simulink model "pid_tv_test2"  (R2016a)
settings: Solver=ode23tb  StartTime=0.0  StopTime=ti(end)  MaxStep=1e-3
InitFcn:
  | fp_sp_k = 12e3;
  | fp_sp_d = 1;
  | weights = 70/6;
  | joint_k = 0*180/pi;
  | joint_d = 0*180/pi;
  | fp_uj_dp_k = 500*180/pi;
  | fp_uj_dp_d = 1*180/pi;
  | fp_uj_ie_k = 500*180/pi;
  | fp_uj_ie_d = 1*180/pi;
values from neighbouring files (symbols this model uses):
  N = length(shin_angles_in.signals.values)    [GaitEmu_code.m]    (also in dy1.m; dy2.m; est_joint.m = size( [body1.trans body2.trans], 1 ); impcont.m)
  s = [-atan((t2.*3.379e-4+t3+t4.*t5.*4.401e-2)./(t4.*cos(q2)));-asin(t2.*1.4870979e-5+t3.*4.401e-2-t4.*t5)]    [FK_af.m]    (also in FK_footimp.m = [atan((ree2_1.*t2.*4.401e-2+ree2_2.*t4+ree2_3.*t3+t5.*t7.*4.; FK_gaitEmul.m = [q1+t2.*t4.*4.234e-1+t3.*t5.*1.5e-3-t2.*t6.*t7.*1.5e-3-5.347; ik.m = [x; y; z]; ik_af.m = FK_af(q))
  sta = [-0.5345 0.03779 -0.0866]    [GaitEmu_code.m]    (also in dy1.m; dy2.m; grn_dyn.m; impcont.m)
  Y = -( reshape( body1.trans', [], 1 ) - reshape( body2.trans', [], 1 ) )    [creat_joint.m]    (also in est_joint.m = -( reshape( body1.trans', [3*N 1] ) - reshape( body2.trans',)
undefined symbols (not defined in the file or in its folder): X, Z
libraries: sm_lib x263, nesl_utility x76, simulink x4, dspstat3 x1
(part 6 of 6)

== system pid_tv_test2/Gait Emulator/prismatic frame1/y_bar_w_weightWalk_Sim1_1_RIGID/weight_4_RIGID ==
  ReferenceFrame : sm_lib/Frames and Transforms/Reference Frame
  Solid : sm_lib/Body Elements/Solid  InertiaType=Custom  Mass=weights  MassUnits=kg  CenterOfMass=[-0.093540130299891208 0.042272178743630776 0.014999999999999999]  CenterOfMassUnits=m  MomentsOfInertia=[0.0088271162208858108 0.0088271162208858108 0.017393538113134353]  MomentsOfInertiaUnits=kg*m^2  ProductsOfInertia=[0 0 0]  ProductsOfInertiaUnits=kg*m^2  DensityBased=on  Density=1000  DensityUnits=kg/(m^3)  DoExposeReferenceFrame=on  SerializedFrames=<Frames/>  GraphicType=FromGeometry  MarkerShape=Sphere  MarkerSize=10  MarkerSizeUnits=m  GraphicVisPropType=SimpleVisualProperties  GraphicDiffuseColor=[0.792156862745098 0.81960784313725488 0.93333333333333335]  GraphicSpecularColor=[0.5 0.5 0.5 1.0]  GraphicAmbientColor=[0.15 0.15 0.15 1.0]  GraphicEmissiveColor=[0.0 0.0 0.0 1.0]  GraphicShininess=75  GraphicOpacity=1  GeometryShape=FromFile  RectangleSize=[1 1]  RectangleSizeUnits=m  BrickDimensions=[1 1 1]  BrickDimensionUnits=m  CylinderRadius=1  CylinderRadiusUnits=m  CylinderLength=1  CylinderLengthUnits=m  SphereRadius=1  SphereRadiusUnits=m  EllipsoidRadii=[1 1 1]  EllipsoidRadiiUnits=m  ExtrusionCrossSection=[1 1; -1 1; -1 -1; 1 -1]  ExtrusionCrossSectionUnits=m  ExtrusionLength=1  ExtrusionLengthUnits=m  PolygonNumSides=3  PolygonOuterRadius=1  PolygonOuterRadiusUnits=m  ExtGeomFileType=STL  ExtGeomFileName=weight_Default_sldprt.STL  ExtGeomFileUnits=m  RevolutionCrossSection=[1 1; 1 -1; 2 -1; 2 1]  RevolutionCrossSectionUnits=m  RevolutionExtent=Full  RevolutionAngle=180  RevolutionAngleUnits=deg
  F : PMIOPort  Port=1  Side=Left
  connections:
  Solid/RConn1 -- ReferenceFrame/RConn1 -- F/RConn1

== system pid_tv_test2/Gait Emulator/prismatic frame1/y_bar_w_weightWalk_Sim1_1_RIGID/weight_5_RIGID ==
  ReferenceFrame : sm_lib/Frames and Transforms/Reference Frame
  Solid : sm_lib/Body Elements/Solid  InertiaType=Custom  Mass=weights  MassUnits=kg  CenterOfMass=[-0.093540130299891208 0.042272178743630776 0.014999999999999999]  CenterOfMassUnits=m  MomentsOfInertia=[0.0088271162208858108 0.0088271162208858108 0.017393538113134353]  MomentsOfInertiaUnits=kg*m^2  ProductsOfInertia=[0 0 0]  ProductsOfInertiaUnits=kg*m^2  DensityBased=on  Density=1000  DensityUnits=kg/(m^3)  DoExposeReferenceFrame=on  SerializedFrames=<Frames/>  GraphicType=FromGeometry  MarkerShape=Sphere  MarkerSize=10  MarkerSizeUnits=m  GraphicVisPropType=SimpleVisualProperties  GraphicDiffuseColor=[0.792156862745098 0.81960784313725488 0.93333333333333335]  GraphicSpecularColor=[0.5 0.5 0.5 1.0]  GraphicAmbientColor=[0.15 0.15 0.15 1.0]  GraphicEmissiveColor=[0.0 0.0 0.0 1.0]  GraphicShininess=75  GraphicOpacity=1  GeometryShape=FromFile  RectangleSize=[1 1]  RectangleSizeUnits=m  BrickDimensions=[1 1 1]  BrickDimensionUnits=m  CylinderRadius=1  CylinderRadiusUnits=m  CylinderLength=1  CylinderLengthUnits=m  SphereRadius=1  SphereRadiusUnits=m  EllipsoidRadii=[1 1 1]  EllipsoidRadiiUnits=m  ExtrusionCrossSection=[1 1; -1 1; -1 -1; 1 -1]  ExtrusionCrossSectionUnits=m  ExtrusionLength=1  ExtrusionLengthUnits=m  PolygonNumSides=3  PolygonOuterRadius=1  PolygonOuterRadiusUnits=m  ExtGeomFileType=STL  ExtGeomFileName=weight_Default_sldprt.STL  ExtGeomFileUnits=m  RevolutionCrossSection=[1 1; 1 -1; 2 -1; 2 1]  RevolutionCrossSectionUnits=m  RevolutionExtent=Full  RevolutionAngle=180  RevolutionAngleUnits=deg
  F : PMIOPort  Port=1  Side=Left
  connections:
  Solid/RConn1 -- ReferenceFrame/RConn1 -- F/RConn1

== system pid_tv_test2/Gait Emulator/prismatic frame1/y_bar_w_weightWalk_Sim1_1_RIGID/weight_6_RIGID ==
  ReferenceFrame : sm_lib/Frames and Transforms/Reference Frame
  Solid : sm_lib/Body Elements/Solid  InertiaType=Custom  Mass=weights  MassUnits=kg  CenterOfMass=[-0.093540130299891208 0.042272178743630776 0.014999999999999999]  CenterOfMassUnits=m  MomentsOfInertia=[0.0088271162208858108 0.0088271162208858108 0.017393538113134353]  MomentsOfInertiaUnits=kg*m^2  ProductsOfInertia=[0 0 0]  ProductsOfInertiaUnits=kg*m^2  DensityBased=on  Density=1000  DensityUnits=kg/(m^3)  DoExposeReferenceFrame=on  SerializedFrames=<Frames/>  GraphicType=FromGeometry  MarkerShape=Sphere  MarkerSize=10  MarkerSizeUnits=m  GraphicVisPropType=SimpleVisualProperties  GraphicDiffuseColor=[0.792156862745098 0.81960784313725488 0.93333333333333335]  GraphicSpecularColor=[0.5 0.5 0.5 1.0]  GraphicAmbientColor=[0.15 0.15 0.15 1.0]  GraphicEmissiveColor=[0.0 0.0 0.0 1.0]  GraphicShininess=75  GraphicOpacity=1  GeometryShape=FromFile  RectangleSize=[1 1]  RectangleSizeUnits=m  BrickDimensions=[1 1 1]  BrickDimensionUnits=m  CylinderRadius=1  CylinderRadiusUnits=m  CylinderLength=1  CylinderLengthUnits=m  SphereRadius=1  SphereRadiusUnits=m  EllipsoidRadii=[1 1 1]  EllipsoidRadiiUnits=m  ExtrusionCrossSection=[1 1; -1 1; -1 -1; 1 -1]  ExtrusionCrossSectionUnits=m  ExtrusionLength=1  ExtrusionLengthUnits=m  PolygonNumSides=3  PolygonOuterRadius=1  PolygonOuterRadiusUnits=m  ExtGeomFileType=STL  ExtGeomFileName=weight_Default_sldprt.STL  ExtGeomFileUnits=m  RevolutionCrossSection=[1 1; 1 -1; 2 -1; 2 1]  RevolutionCrossSectionUnits=m  RevolutionExtent=Full  RevolutionAngle=180  RevolutionAngleUnits=deg
  F : PMIOPort  Port=1  Side=Left
  connections:
  Solid/RConn1 -- ReferenceFrame/RConn1 -- F/RConn1

== system pid_tv_test2/Gait Emulator/prismatic frame1/y_bar_w_weightWalk_Sim1_1_RIGID/y_bar_1_RIGID ==
  ReferenceFrame : sm_lib/Frames and Transforms/Reference Frame
  Solid : sm_lib/Body Elements/Solid  InertiaType=Custom  Mass=0.47799554976271263  MassUnits=kg  CenterOfMass=[0.00076616175672379865 -0.25377093214757318 3.5664030409292288e-05]  CenterOfMassUnits=m  MomentsOfInertia=[0.010298158029361381 7.4602586681976561e-05 0.010304194450422657]  MomentsOfInertiaUnits=kg*m^2  ProductsOfInertia=[-6.4284014840620861e-08 -2.8526588755049515e-07 -1.380997973988322e-06]  ProductsOfInertiaUnits=kg*m^2  DensityBased=on  Density=1000  DensityUnits=kg/(m^3)  DoExposeReferenceFrame=on  SerializedFrames=<Frames/>  GraphicType=FromGeometry  MarkerShape=Sphere  MarkerSize=10  MarkerSizeUnits=m  GraphicVisPropType=SimpleVisualProperties  GraphicDiffuseColor=[1.0 0.0 0.2]  GraphicSpecularColor=[0.5 0.5 0.5 1.0]  GraphicAmbientColor=[0.15 0.15 0.15 1.0]  GraphicEmissiveColor=[0.0 0.0 0.0 1.0]  GraphicShininess=75  GraphicOpacity=1  GeometryShape=FromFile  RectangleSize=[1 1]  RectangleSizeUnits=m  BrickDimensions=[1 1 1]  BrickDimensionUnits=m  CylinderRadius=1  CylinderRadiusUnits=m  CylinderLength=1  CylinderLengthUnits=m  SphereRadius=1  SphereRadiusUnits=m  EllipsoidRadii=[1 1 1]  EllipsoidRadiiUnits=m  ExtrusionCrossSection=[1 1; -1 1; -1 -1; 1 -1]  ExtrusionCrossSectionUnits=m  ExtrusionLength=1  ExtrusionLengthUnits=m  PolygonNumSides=3  PolygonOuterRadius=1  PolygonOuterRadiusUnits=m  ExtGeomFileType=STL  ExtGeomFileName=y_bar_Default_sldprt.STL  ExtGeomFileUnits=m  RevolutionCrossSection=[1 1; 1 -1; 2 -1; 2 1]  RevolutionCrossSectionUnits=m  RevolutionExtent=Full  RevolutionAngle=180  RevolutionAngleUnits=deg
  F : PMIOPort  Port=1  Side=Left
  connections:
  Solid/RConn1 -- ReferenceFrame/RConn1 -- F/RConn1

== system pid_tv_test2/Gait Emulator/Walkway & force plate/Force Plate/base_frame_1_RIGID/x8020_1020_1020_X_50cm_1_RIGID ==
  ReferenceFrame : sm_lib/Frames and Transforms/Reference Frame
  Solid : sm_lib/Body Elements/Solid  InertiaType=Custom  Mass=0.25907382645160842  MassUnits=kg  CenterOfMass=[0 0 0]  CenterOfMassUnits=in  MomentsOfInertia=[8.3933307234335093 8.4665424365077708 0.12805533197749852]  MomentsOfInertiaUnits=kg*in^2  ProductsOfInertia=[0 0 0]  ProductsOfInertiaUnits=kg*in^2  DensityBased=on  Density=1000  DensityUnits=kg/(m^3)  DoExposeReferenceFrame=on  SerializedFrames=<Frames/>  GraphicType=FromGeometry  MarkerShape=Sphere  MarkerSize=10  MarkerSizeUnits=m  GraphicVisPropType=SimpleVisualProperties  GraphicDiffuseColor=[1 1 1]  GraphicSpecularColor=[0.5 0.5 0.5 1.0]  GraphicAmbientColor=[0.15 0.15 0.15 1.0]  GraphicEmissiveColor=[0.0 0.0 0.0 1.0]  GraphicShininess=75  GraphicOpacity=1  GeometryShape=FromFile  RectangleSize=[1 1]  RectangleSizeUnits=m  BrickDimensions=[1 1 1]  BrickDimensionUnits=m  CylinderRadius=1  CylinderRadiusUnits=m  CylinderLength=1  CylinderLengthUnits=m  SphereRadius=1  SphereRadiusUnits=m  EllipsoidRadii=[1 1 1]  EllipsoidRadiiUnits=m  ExtrusionCrossSection=[1 1; -1 1; -1 -1; 1 -1]  ExtrusionCrossSectionUnits=m  ExtrusionLength=1  ExtrusionLengthUnits=m  PolygonNumSides=3  PolygonOuterRadius=1  PolygonOuterRadiusUnits=m  ExtGeomFileType=STL  ExtGeomFileName=8020-1020-1020 X 50cm_Default_sldprt.STL  ExtGeomFileUnits=in  RevolutionCrossSection=[1 1; 1 -1; 2 -1; 2 1]  RevolutionCrossSectionUnits=m  RevolutionExtent=Full  RevolutionAngle=180  RevolutionAngleUnits=deg
  F : PMIOPort  Port=1  Side=Left
  connections:
  ReferenceFrame/RConn1 -- Solid/RConn1 -- F/RConn1

== system pid_tv_test2/Gait Emulator/Walkway & force plate/Force Plate/base_frame_1_RIGID/x8020_1020_1020_X_50cm_2_RIGID ==
  ReferenceFrame : sm_lib/Frames and Transforms/Reference Frame
  Solid : sm_lib/Body Elements/Solid  InertiaType=Custom  Mass=0.25907382645160842  MassUnits=kg  CenterOfMass=[0 0 0]  CenterOfMassUnits=in  MomentsOfInertia=[8.3933307234335093 8.4665424365077708 0.12805533197749852]  MomentsOfInertiaUnits=kg*in^2  ProductsOfInertia=[0 0 0]  ProductsOfInertiaUnits=kg*in^2  DensityBased=on  Density=1000  DensityUnits=kg/(m^3)  DoExposeReferenceFrame=on  SerializedFrames=<Frames/>  GraphicType=FromGeometry  MarkerShape=Sphere  MarkerSize=10  MarkerSizeUnits=m  GraphicVisPropType=SimpleVisualProperties  GraphicDiffuseColor=[1 1 1]  GraphicSpecularColor=[0.5 0.5 0.5 1.0]  GraphicAmbientColor=[0.15 0.15 0.15 1.0]  GraphicEmissiveColor=[0.0 0.0 0.0 1.0]  GraphicShininess=75  GraphicOpacity=1  GeometryShape=FromFile  RectangleSize=[1 1]  RectangleSizeUnits=m  BrickDimensions=[1 1 1]  BrickDimensionUnits=m  CylinderRadius=1  CylinderRadiusUnits=m  CylinderLength=1  CylinderLengthUnits=m  SphereRadius=1  SphereRadiusUnits=m  EllipsoidRadii=[1 1 1]  EllipsoidRadiiUnits=m  ExtrusionCrossSection=[1 1; -1 1; -1 -1; 1 -1]  ExtrusionCrossSectionUnits=m  ExtrusionLength=1  ExtrusionLengthUnits=m  PolygonNumSides=3  PolygonOuterRadius=1  PolygonOuterRadiusUnits=m  ExtGeomFileType=STL  ExtGeomFileName=8020-1020-1020 X 50cm_Default_sldprt.STL  ExtGeomFileUnits=in  RevolutionCrossSection=[1 1; 1 -1; 2 -1; 2 1]  RevolutionCrossSectionUnits=m  RevolutionExtent=Full  RevolutionAngle=180  RevolutionAngleUnits=deg
  F : PMIOPort  Port=1  Side=Left
  connections:
  ReferenceFrame/RConn1 -- Solid/RConn1 -- F/RConn1

== system pid_tv_test2/Gait Emulator/Walkway & force plate/Force Plate/base_frame_1_RIGID/x8020_1020_1020_X_7_81_1_RIGID ==
  ReferenceFrame : sm_lib/Frames and Transforms/Reference Frame
  Solid : sm_lib/Body Elements/Solid  InertiaType=Custom  Mass=0.10278722807147889  MassUnits=kg  CenterOfMass=[0 0 0]  CenterOfMassUnits=in  MomentsOfInertia=[0.53334790666301179 0.56239456549511713 0.050805798463005557]  MomentsOfInertiaUnits=kg*in^2  ProductsOfInertia=[0 0 0]  ProductsOfInertiaUnits=kg*in^2  DensityBased=on  Density=1000  DensityUnits=kg/(m^3)  DoExposeReferenceFrame=on  SerializedFrames=<Frames/>  GraphicType=FromGeometry  MarkerShape=Sphere  MarkerSize=10  MarkerSizeUnits=m  GraphicVisPropType=SimpleVisualProperties  GraphicDiffuseColor=[1 1 1]  GraphicSpecularColor=[0.5 0.5 0.5 1.0]  GraphicAmbientColor=[0.15 0.15 0.15 1.0]  GraphicEmissiveColor=[0.0 0.0 0.0 1.0]  GraphicShininess=75  GraphicOpacity=1  GeometryShape=FromFile  RectangleSize=[1 1]  RectangleSizeUnits=m  BrickDimensions=[1 1 1]  BrickDimensionUnits=m  CylinderRadius=1  CylinderRadiusUnits=m  CylinderLength=1  CylinderLengthUnits=m  SphereRadius=1  SphereRadiusUnits=m  EllipsoidRadii=[1 1 1]  EllipsoidRadiiUnits=m  ExtrusionCrossSection=[1 1; -1 1; -1 -1; 1 -1]  ExtrusionCrossSectionUnits=m  ExtrusionLength=1  ExtrusionLengthUnits=m  PolygonNumSides=3  PolygonOuterRadius=1  PolygonOuterRadiusUnits=m  ExtGeomFileType=STL  ExtGeomFileName=8020-1020-1020 X 7_81_Default_sldprt.STL  ExtGeomFileUnits=in  RevolutionCrossSection=[1 1; 1 -1; 2 -1; 2 1]  RevolutionCrossSectionUnits=m  RevolutionExtent=Full  RevolutionAngle=180  RevolutionAngleUnits=deg
  F : PMIOPort  Port=1  Side=Left
  connections:
  ReferenceFrame/RConn1 -- Solid/RConn1 -- F/RConn1

== system pid_tv_test2/Gait Emulator/Walkway & force plate/Force Plate/base_frame_1_RIGID/x8020_1020_1020_X_7_81_2_RIGID ==
  ReferenceFrame : sm_lib/Frames and Transforms/Reference Frame
  Solid : sm_lib/Body Elements/Solid  InertiaType=Custom  Mass=0.10278722807147889  MassUnits=kg  CenterOfMass=[0 0 0]  CenterOfMassUnits=in  MomentsOfInertia=[0.53334790666301179 0.56239456549511713 0.050805798463005557]  MomentsOfInertiaUnits=kg*in^2  ProductsOfInertia=[0 0 0]  ProductsOfInertiaUnits=kg*in^2  DensityBased=on  Density=1000  DensityUnits=kg/(m^3)  DoExposeReferenceFrame=on  SerializedFrames=<Frames/>  GraphicType=FromGeometry  MarkerShape=Sphere  MarkerSize=10  MarkerSizeUnits=m  GraphicVisPropType=SimpleVisualProperties  GraphicDiffuseColor=[1 1 1]  GraphicSpecularColor=[0.5 0.5 0.5 1.0]  GraphicAmbientColor=[0.15 0.15 0.15 1.0]  GraphicEmissiveColor=[0.0 0.0 0.0 1.0]  GraphicShininess=75  GraphicOpacity=1  GeometryShape=FromFile  RectangleSize=[1 1]  RectangleSizeUnits=m  BrickDimensions=[1 1 1]  BrickDimensionUnits=m  CylinderRadius=1  CylinderRadiusUnits=m  CylinderLength=1  CylinderLengthUnits=m  SphereRadius=1  SphereRadiusUnits=m  EllipsoidRadii=[1 1 1]  EllipsoidRadiiUnits=m  ExtrusionCrossSection=[1 1; -1 1; -1 -1; 1 -1]  ExtrusionCrossSectionUnits=m  ExtrusionLength=1  ExtrusionLengthUnits=m  PolygonNumSides=3  PolygonOuterRadius=1  PolygonOuterRadiusUnits=m  ExtGeomFileType=STL  ExtGeomFileName=8020-1020-1020 X 7_81_Default_sldprt.STL  ExtGeomFileUnits=in  RevolutionCrossSection=[1 1; 1 -1; 2 -1; 2 1]  RevolutionCrossSectionUnits=m  RevolutionExtent=Full  RevolutionAngle=180  RevolutionAngleUnits=deg
  F : PMIOPort  Port=1  Side=Left
  connections:
  ReferenceFrame/RConn1 -- Solid/RConn1 -- F/RConn1

== system pid_tv_test2/Gait Emulator/Walkway & force plate/Force Plate/base_frame_1_RIGID/x8020_1020_1020_X_7_81_3_RIGID ==
  ReferenceFrame : sm_lib/Frames and Transforms/Reference Frame
  Solid : sm_lib/Body Elements/Solid  InertiaType=Custom  Mass=0.10278722807147889  MassUnits=kg  CenterOfMass=[0 0 0]  CenterOfMassUnits=in  MomentsOfInertia=[0.53334790666301179 0.56239456549511713 0.050805798463005557]  MomentsOfInertiaUnits=kg*in^2  ProductsOfInertia=[0 0 0]  ProductsOfInertiaUnits=kg*in^2  DensityBased=on  Density=1000  DensityUnits=kg/(m^3)  DoExposeReferenceFrame=on  SerializedFrames=<Frames/>  GraphicType=FromGeometry  MarkerShape=Sphere  MarkerSize=10  MarkerSizeUnits=m  GraphicVisPropType=SimpleVisualProperties  GraphicDiffuseColor=[1 1 1]  GraphicSpecularColor=[0.5 0.5 0.5 1.0]  GraphicAmbientColor=[0.15 0.15 0.15 1.0]  GraphicEmissiveColor=[0.0 0.0 0.0 1.0]  GraphicShininess=75  GraphicOpacity=1  GeometryShape=FromFile  RectangleSize=[1 1]  RectangleSizeUnits=m  BrickDimensions=[1 1 1]  BrickDimensionUnits=m  CylinderRadius=1  CylinderRadiusUnits=m  CylinderLength=1  CylinderLengthUnits=m  SphereRadius=1  SphereRadiusUnits=m  EllipsoidRadii=[1 1 1]  EllipsoidRadiiUnits=m  ExtrusionCrossSection=[1 1; -1 1; -1 -1; 1 -1]  ExtrusionCrossSectionUnits=m  ExtrusionLength=1  ExtrusionLengthUnits=m  PolygonNumSides=3  PolygonOuterRadius=1  PolygonOuterRadiusUnits=m  ExtGeomFileType=STL  ExtGeomFileName=8020-1020-1020 X 7_81_Default_sldprt.STL  ExtGeomFileUnits=in  RevolutionCrossSection=[1 1; 1 -1; 2 -1; 2 1]  RevolutionCrossSectionUnits=m  RevolutionExtent=Full  RevolutionAngle=180  RevolutionAngleUnits=deg
  F : PMIOPort  Port=1  Side=Left
  connections:
  ReferenceFrame/RConn1 -- Solid/RConn1 -- F/RConn1

== system pid_tv_test2/Gait Emulator/Walkway & force plate/Force Plate/top_frame_1_RIGID/frame1_1_RIGID ==
  ReferenceFrame : sm_lib/Frames and Transforms/Reference Frame
  Transform : sm_lib/Frames and Transforms/Rigid Transform  TranslationMethod=Cartesian  TranslationLengthUnit=m  TranslationStandardAxis=+Z  TranslationStandardOffset=0  TranslationCartesianOffset=[0.099187000000000025 -1.27675647831893e-15 -0.24999950000000001]  TranslationROffset=0  TranslationROffsetUnits=m  TranslationZOffset=0  TranslationZOffsetUnits=m  TranslationThetaOffset=0  TranslationThetaOffsetUnits=deg  RotationMethod=None  RotationAngleUnits=deg  RotationStandardAxis=+Z  RotationAngle=0.0  RotationArbitraryAxis=[0 0 1]  FollAlignAxisA=+X  BaseAlignAxisA=+Y  FollAlignAxisB=+Y  BaseAlignAxisB=+Z  RotationSequenceAxes=FollowerAxes  RotationSequence=XYX  RotationSequenceAngles=[0 0 0]  RotationSequenceAnglesUnits=deg  RotationMatrix=[1 0 0; 0 1 0; 0 0 1]
  Transform1 : sm_lib/Frames and Transforms/Rigid Transform  TranslationMethod=Cartesian  TranslationLengthUnit=m  TranslationStandardAxis=+Z  TranslationStandardOffset=0  TranslationCartesianOffset=[0.22377399999999997 0 -0.47459899999999999]  TranslationROffset=0  TranslationROffsetUnits=m  TranslationZOffset=0  TranslationZOffsetUnits=m  TranslationThetaOffset=0  TranslationThetaOffsetUnits=deg  RotationMethod=ArbitraryAxis  RotationAngleUnits=rad  RotationStandardAxis=+Z  RotationAngle=1.5707963267948968  RotationArbitraryAxis=[2.10991883731723e-15 1 5.8442032848726394e-16]  FollAlignAxisA=+X  BaseAlignAxisA=+Y  FollAlignAxisB=+Y  BaseAlignAxisB=+Z  RotationSequenceAxes=FollowerAxes  RotationSequence=XYX  RotationSequenceAngles=[0 0 0]  RotationSequenceAnglesUnits=deg  RotationMatrix=[1 0 0; 0 1 0; 0 0 1]
  Transform2 : sm_lib/Frames and Transforms/Rigid Transform  TranslationMethod=Cartesian  TranslationLengthUnit=m  TranslationStandardAxis=+Z  TranslationStandardOffset=0  TranslationCartesianOffset=[0.34836099999999992 -2.400857290751901e-15 -0.24999950000000001]  TranslationROffset=0  TranslationROffsetUnits=m  TranslationZOffset=0  TranslationZOffsetUnits=m  TranslationThetaOffset=0  TranslationThetaOffsetUnits=deg  RotationMethod=ArbitraryAxis  RotationAngleUnits=rad  RotationStandardAxis=+Z  RotationAngle=3.1415926535897931  RotationArbitraryAxis=[1.2403272853234171e-15 1 -5.0658111711395872e-16]  FollAlignAxisA=+X  BaseAlignAxisA=+Y  FollAlignAxisB=+Y  BaseAlignAxisB=+Z  RotationSequenceAxes=FollowerAxes  RotationSequence=XYX  RotationSequenceAngles=[0 0 0]  RotationSequenceAnglesUnits=deg  RotationMatrix=[1 0 0; 0 1 0; 0 0 1]
  Transform3 : sm_lib/Frames and Transforms/Rigid Transform  TranslationMethod=Cartesian  TranslationLengthUnit=m  TranslationStandardAxis=+Z  TranslationStandardOffset=0  TranslationCartesianOffset=[0.22377399999999986 -1.3322676295501878e-15 -0.025400000000000061]  TranslationROffset=0  TranslationROffsetUnits=m  TranslationZOffset=0  TranslationZOffsetUnits=m  TranslationThetaOffset=0  TranslationThetaOffsetUnits=deg  RotationMethod=ArbitraryAxis  RotationAngleUnits=rad  RotationStandardAxis=+Z  RotationAngle=1.5707963267948968  RotationArbitraryAxis=[-4.7691944979696082e-15 -1 -6.6899476726480988e-16]  FollAlignAxisA=+X  BaseAlignAxisA=+Y  FollAlignAxisB=+Y  BaseAlignAxisB=+Z  RotationSequenceAxes=FollowerAxes  RotationSequence=XYX  RotationSequenceAngles=[0 0 0]  RotationSequenceAnglesUnits=deg  RotationMatrix=[1 0 0; 0 1 0; 0 0 1]
  Transform4 : sm_lib/Frames and Transforms/Rigid Transform  TranslationMethod=Cartesian  TranslationLengthUnit=m  TranslationStandardAxis=+Z  TranslationStandardOffset=0  TranslationCartesianOffset=[-0.24999899999999994 0.025400000000001838 -0.22377400000000008]  TranslationROffset=0  TranslationROffsetUnits=m  TranslationZOffset=0  TranslationZOffsetUnits=m  TranslationThetaOffset=0  TranslationThetaOffsetUnits=deg  RotationMethod=ArbitraryAxis  RotationAngleUnits=rad  RotationStandardAxis=+Z  RotationAngle=1.5707963267948968  RotationArbitraryAxis=[-3.5952694497400173e-15 -1 1.7432631046654889e-15]  FollAlignAxisA=+X  BaseAlignAxisA=+Y  FollAlignAxisB=+Y  BaseAlignAxisB=+Z  RotationSequenceAxes=FollowerAxes  RotationSequence=XYX  RotationSequenceAngles=[0 0 0]  RotationSequenceAnglesUnits=deg  RotationMatrix=[1 0 0; 0 1 0; 0 0 1]
  x8020_1020_1020_X_50cm_1_RIGID : Subsystem
  x8020_1020_1020_X_50cm_2_RIGID : Subsystem
  x8020_1020_1020_X_7_81_1_RIGID : Subsystem
  x8020_1020_1020_X_7_81_2_RIGID : Subsystem
  F : PMIOPort  Port=1  Side=Right
  connections:
  Transform/RConn1 -- x8020_1020_1020_X_50cm_1_RIGID/LConn1
  Transform1/RConn1 -- x8020_1020_1020_X_7_81_1_RIGID/LConn1
  Transform2/RConn1 -- x8020_1020_1020_X_50cm_2_RIGID/LConn1
  Transform3/RConn1 -- x8020_1020_1020_X_7_81_2_RIGID/LConn1
  ReferenceFrame/RConn1 -- Transform2/LConn1 -- Transform3/LConn1 -- Transform/LConn1 -- Transform1/LConn1 -- Transform4/RConn1
  Transform4/LConn1 -- F/RConn1

== system pid_tv_test2/Gait Emulator/Walkway & force plate/Force Plate/top_frame_1_RIGID/x8020_1020_1020_X_11_81_1_RIGID ==
  ReferenceFrame : sm_lib/Frames and Transforms/Reference Frame
  Solid : sm_lib/Body Elements/Solid  InertiaType=Custom  Mass=0.15543113489425955  MassUnits=kg  CenterOfMass=[0 0 0]  CenterOfMassUnits=in  MomentsOfInertia=[1.8230290687756983 1.8669523774577936 0.076826693962624301]  MomentsOfInertiaUnits=kg*in^2  ProductsOfInertia=[0 0 0]  ProductsOfInertiaUnits=kg*in^2  DensityBased=on  Density=1000  DensityUnits=kg/(m^3)  DoExposeReferenceFrame=on  SerializedFrames=<Frames/>  GraphicType=FromGeometry  MarkerShape=Sphere  MarkerSize=10  MarkerSizeUnits=m  GraphicVisPropType=SimpleVisualProperties  GraphicDiffuseColor=[1 1 1]  GraphicSpecularColor=[0.5 0.5 0.5 1.0]  GraphicAmbientColor=[0.15 0.15 0.15 1.0]  GraphicEmissiveColor=[0.0 0.0 0.0 1.0]  GraphicShininess=75  GraphicOpacity=1  GeometryShape=FromFile  RectangleSize=[1 1]  RectangleSizeUnits=m  BrickDimensions=[1 1 1]  BrickDimensionUnits=m  CylinderRadius=1  CylinderRadiusUnits=m  CylinderLength=1  CylinderLengthUnits=m  SphereRadius=1  SphereRadiusUnits=m  EllipsoidRadii=[1 1 1]  EllipsoidRadiiUnits=m  ExtrusionCrossSection=[1 1; -1 1; -1 -1; 1 -1]  ExtrusionCrossSectionUnits=m  ExtrusionLength=1  ExtrusionLengthUnits=m  PolygonNumSides=3  PolygonOuterRadius=1  PolygonOuterRadiusUnits=m  ExtGeomFileType=STL  ExtGeomFileName=8020-1020-1020 X 11_81_Default_sldprt.STL  ExtGeomFileUnits=in  RevolutionCrossSection=[1 1; 1 -1; 2 -1; 2 1]  RevolutionCrossSectionUnits=m  RevolutionExtent=Full  RevolutionAngle=180  RevolutionAngleUnits=deg
  F : PMIOPort  Port=1  Side=Left
  connections:
  ReferenceFrame/RConn1 -- Solid/RConn1 -- F/RConn1

== system pid_tv_test2/Gait Emulator/Walkway & force plate/Force Plate/top_frame_1_RIGID/frame1_1_RIGID/x8020_1020_1020_X_50cm_1_RIGID ==
  ReferenceFrame : sm_lib/Frames and Transforms/Reference Frame
  Solid : sm_lib/Body Elements/Solid  InertiaType=Custom  Mass=0.25907382645160842  MassUnits=kg  CenterOfMass=[0 0 0]  CenterOfMassUnits=in  MomentsOfInertia=[8.3933307234335093 8.4665424365077708 0.12805533197749852]  MomentsOfInertiaUnits=kg*in^2  ProductsOfInertia=[0 0 0]  ProductsOfInertiaUnits=kg*in^2  DensityBased=on  Density=1000  DensityUnits=kg/(m^3)  DoExposeReferenceFrame=on  SerializedFrames=<Frames/>  GraphicType=FromGeometry  MarkerShape=Sphere  MarkerSize=10  MarkerSizeUnits=m  GraphicVisPropType=SimpleVisualProperties  GraphicDiffuseColor=[1 1 1]  GraphicSpecularColor=[0.5 0.5 0.5 1.0]  GraphicAmbientColor=[0.15 0.15 0.15 1.0]  GraphicEmissiveColor=[0.0 0.0 0.0 1.0]  GraphicShininess=75  GraphicOpacity=1  GeometryShape=FromFile  RectangleSize=[1 1]  RectangleSizeUnits=m  BrickDimensions=[1 1 1]  BrickDimensionUnits=m  CylinderRadius=1  CylinderRadiusUnits=m  CylinderLength=1  CylinderLengthUnits=m  SphereRadius=1  SphereRadiusUnits=m  EllipsoidRadii=[1 1 1]  EllipsoidRadiiUnits=m  ExtrusionCrossSection=[1 1; -1 1; -1 -1; 1 -1]  ExtrusionCrossSectionUnits=m  ExtrusionLength=1  ExtrusionLengthUnits=m  PolygonNumSides=3  PolygonOuterRadius=1  PolygonOuterRadiusUnits=m  ExtGeomFileType=STL  ExtGeomFileName=8020-1020-1020 X 50cm_Default_sldprt.STL  ExtGeomFileUnits=in  RevolutionCrossSection=[1 1; 1 -1; 2 -1; 2 1]  RevolutionCrossSectionUnits=m  RevolutionExtent=Full  RevolutionAngle=180  RevolutionAngleUnits=deg
  F : PMIOPort  Port=1  Side=Left
  connections:
  ReferenceFrame/RConn1 -- Solid/RConn1 -- F/RConn1

== system pid_tv_test2/Gait Emulator/Walkway & force plate/Force Plate/top_frame_1_RIGID/frame1_1_RIGID/x8020_1020_1020_X_50cm_2_RIGID ==
  ReferenceFrame : sm_lib/Frames and Transforms/Reference Frame
  Solid : sm_lib/Body Elements/Solid  InertiaType=Custom  Mass=0.25907382645160842  MassUnits=kg  CenterOfMass=[0 0 0]  CenterOfMassUnits=in  MomentsOfInertia=[8.3933307234335093 8.4665424365077708 0.12805533197749852]  MomentsOfInertiaUnits=kg*in^2  ProductsOfInertia=[0 0 0]  ProductsOfInertiaUnits=kg*in^2  DensityBased=on  Density=1000  DensityUnits=kg/(m^3)  DoExposeReferenceFrame=on  SerializedFrames=<Frames/>  GraphicType=FromGeometry  MarkerShape=Sphere  MarkerSize=10  MarkerSizeUnits=m  GraphicVisPropType=SimpleVisualProperties  GraphicDiffuseColor=[1 1 1]  GraphicSpecularColor=[0.5 0.5 0.5 1.0]  GraphicAmbientColor=[0.15 0.15 0.15 1.0]  GraphicEmissiveColor=[0.0 0.0 0.0 1.0]  GraphicShininess=75  GraphicOpacity=1  GeometryShape=FromFile  RectangleSize=[1 1]  RectangleSizeUnits=m  BrickDimensions=[1 1 1]  BrickDimensionUnits=m  CylinderRadius=1  CylinderRadiusUnits=m  CylinderLength=1  CylinderLengthUnits=m  SphereRadius=1  SphereRadiusUnits=m  EllipsoidRadii=[1 1 1]  EllipsoidRadiiUnits=m  ExtrusionCrossSection=[1 1; -1 1; -1 -1; 1 -1]  ExtrusionCrossSectionUnits=m  ExtrusionLength=1  ExtrusionLengthUnits=m  PolygonNumSides=3  PolygonOuterRadius=1  PolygonOuterRadiusUnits=m  ExtGeomFileType=STL  ExtGeomFileName=8020-1020-1020 X 50cm_Default_sldprt.STL  ExtGeomFileUnits=in  RevolutionCrossSection=[1 1; 1 -1; 2 -1; 2 1]  RevolutionCrossSectionUnits=m  RevolutionExtent=Full  RevolutionAngle=180  RevolutionAngleUnits=deg
  F : PMIOPort  Port=1  Side=Left
  connections:
  ReferenceFrame/RConn1 -- Solid/RConn1 -- F/RConn1

== system pid_tv_test2/Gait Emulator/Walkway & force plate/Force Plate/top_frame_1_RIGID/frame1_1_RIGID/x8020_1020_1020_X_7_81_1_RIGID ==
  ReferenceFrame : sm_lib/Frames and Transforms/Reference Frame
  Solid : sm_lib/Body Elements/Solid  InertiaType=Custom  Mass=0.10278722807147889  MassUnits=kg  CenterOfMass=[0 0 0]  CenterOfMassUnits=in  MomentsOfInertia=[0.53334790666301179 0.56239456549511713 0.050805798463005557]  MomentsOfInertiaUnits=kg*in^2  ProductsOfInertia=[0 0 0]  ProductsOfInertiaUnits=kg*in^2  DensityBased=on  Density=1000  DensityUnits=kg/(m^3)  DoExposeReferenceFrame=on  SerializedFrames=<Frames/>  GraphicType=FromGeometry  MarkerShape=Sphere  MarkerSize=10  MarkerSizeUnits=m  GraphicVisPropType=SimpleVisualProperties  GraphicDiffuseColor=[1 1 1]  GraphicSpecularColor=[0.5 0.5 0.5 1.0]  GraphicAmbientColor=[0.15 0.15 0.15 1.0]  GraphicEmissiveColor=[0.0 0.0 0.0 1.0]  GraphicShininess=75  GraphicOpacity=1  GeometryShape=FromFile  RectangleSize=[1 1]  RectangleSizeUnits=m  BrickDimensions=[1 1 1]  BrickDimensionUnits=m  CylinderRadius=1  CylinderRadiusUnits=m  CylinderLength=1  CylinderLengthUnits=m  SphereRadius=1  SphereRadiusUnits=m  EllipsoidRadii=[1 1 1]  EllipsoidRadiiUnits=m  ExtrusionCrossSection=[1 1; -1 1; -1 -1; 1 -1]  ExtrusionCrossSectionUnits=m  ExtrusionLength=1  ExtrusionLengthUnits=m  PolygonNumSides=3  PolygonOuterRadius=1  PolygonOuterRadiusUnits=m  ExtGeomFileType=STL  ExtGeomFileName=8020-1020-1020 X 7_81_Default_sldprt.STL  ExtGeomFileUnits=in  RevolutionCrossSection=[1 1; 1 -1; 2 -1; 2 1]  RevolutionCrossSectionUnits=m  RevolutionExtent=Full  RevolutionAngle=180  RevolutionAngleUnits=deg
  F : PMIOPort  Port=1  Side=Left
  connections:
  ReferenceFrame/RConn1 -- Solid/RConn1 -- F/RConn1

== system pid_tv_test2/Gait Emulator/Walkway & force plate/Force Plate/top_frame_1_RIGID/frame1_1_RIGID/x8020_1020_1020_X_7_81_2_RIGID ==
  ReferenceFrame : sm_lib/Frames and Transforms/Reference Frame
  Solid : sm_lib/Body Elements/Solid  InertiaType=Custom  Mass=0.10278722807147889  MassUnits=kg  CenterOfMass=[0 0 0]  CenterOfMassUnits=in  MomentsOfInertia=[0.53334790666301179 0.56239456549511713 0.050805798463005557]  MomentsOfInertiaUnits=kg*in^2  ProductsOfInertia=[0 0 0]  ProductsOfInertiaUnits=kg*in^2  DensityBased=on  Density=1000  DensityUnits=kg/(m^3)  DoExposeReferenceFrame=on  SerializedFrames=<Frames/>  GraphicType=FromGeometry  MarkerShape=Sphere  MarkerSize=10  MarkerSizeUnits=m  GraphicVisPropType=SimpleVisualProperties  GraphicDiffuseColor=[1 1 1]  GraphicSpecularColor=[0.5 0.5 0.5 1.0]  GraphicAmbientColor=[0.15 0.15 0.15 1.0]  GraphicEmissiveColor=[0.0 0.0 0.0 1.0]  GraphicShininess=75  GraphicOpacity=1  GeometryShape=FromFile  RectangleSize=[1 1]  RectangleSizeUnits=m  BrickDimensions=[1 1 1]  BrickDimensionUnits=m  CylinderRadius=1  CylinderRadiusUnits=m  CylinderLength=1  CylinderLengthUnits=m  SphereRadius=1  SphereRadiusUnits=m  EllipsoidRadii=[1 1 1]  EllipsoidRadiiUnits=m  ExtrusionCrossSection=[1 1; -1 1; -1 -1; 1 -1]  ExtrusionCrossSectionUnits=m  ExtrusionLength=1  ExtrusionLengthUnits=m  PolygonNumSides=3  PolygonOuterRadius=1  PolygonOuterRadiusUnits=m  ExtGeomFileType=STL  ExtGeomFileName=8020-1020-1020 X 7_81_Default_sldprt.STL  ExtGeomFileUnits=in  RevolutionCrossSection=[1 1; 1 -1; 2 -1; 2 1]  RevolutionCrossSectionUnits=m  RevolutionExtent=Full  RevolutionAngle=180  RevolutionAngleUnits=deg
  F : PMIOPort  Port=1  Side=Left
  connections:
  ReferenceFrame/RConn1 -- Solid/RConn1 -- F/RConn1

== matlab function pid_tv_test2/Gait Emulator/Walkway & force plate/Ground Contact/MATLAB Function ==
  data: p input; F output; v input; Q input; w input; T output
function [F, T] = fcn(p, v, Q, w)
%#codegen

if abs(p(1))>0.25

% R = quat2dcm(Q);
R = [1 - 2*Q(3)^2 - 2*Q(4)^2	2*Q(2)*Q(3) - 2*Q(4)*Q(1)	2*Q(2)*Q(4) + 2*Q(3)*Q(1)
     2*Q(2)*Q(3) + 2*Q(4)*Q(1)	1 - 2*Q(2)^2 - 2*Q(4)^2	2*Q(3)*Q(4) - 2*Q(2)*Q(1)
     2*Q(2)*Q(4) - 2*Q(3)*Q(1)	2*Q(3)*Q(4) + 2*Q(2)*Q(1)	1 - 2*Q(2)^2 - 2*Q(3)^2];

th1 = linspace(-pi/2,pi/2,5);
% th1 = -pi/2 : 0.7 : pi/2;
r1 = 47e-3.*[cos(th1) cos(th1); sin(th1) sin(th1); zeros(size(th1)), zeros(size(th1))]; % circle
th2 = linspace(pi/2,-pi/2,5);
% th2 = pi/2 : -0.7 : -pi/2;
r2 = 47e-3.*[-cos(th2) -cos(th2); sin(th2) sin(th2); zeros(size(th2)), zeros(size(th2))]; % circle
r2(1,:) = bsxfun(@minus,r2(1,:),134e-3);
% r = ([1 1 1; 1 1 -1; 1 -1 1; 1 -1 -1; -1 1 1; -1 1 -1; -1 -1 1; -1 -1 -1].*repmat([0.2 0.1 0],8,1).*0.5).';
% xx = linspace(-0.11,-0.03,2);
xx = -0.07;
% xx = -0.12:0.04:-0.02;
r3 = [repmat(xx,1,2);repmat(47e-3,1,length(xx)),repmat(-47e-3,1,length(xx));zeros(1,size(xx,2)*2)];
r = [r1,r2,r3];

% spring-damper contact modelc
K = [0 0 0; 0 0 0; 0 0 10]*2e4;
B = [10 0 0; 0 10 0; 0 0 10]*2e2;
% K = [0 0 0; 0 0 0; 0 0 1]*2e3;
% B = [1 0 0; 0 1 0; 0 0 1]*2e2;

rr = bsxfun(@plus, R*r, p); % vertex position on base frame
vv = bsxfun(@plus, v, bsxfun(@cross, w, R*r)); % vertex velocity on base frame

FF = -K*(rr - 0) - B*vv; % force on vertex on base frame

% point is active if normal force is compressing ground
loss = 1 ./ ( 1 + exp(-[0 0 1]*FF) );
% loss = 1 ./ ( 1 + exp(150*[0 0 1]*rr) );

% displace force to coordinate center

% if abs(p(1))>=0.15 && abs(p(2))>=0.1
%     F=[0 0 0]';
%     T=[0 0 0]';
% else
    F = sum( repmat(loss,[3 1]) .* FF, 2 ); % contact force on base frame
    T = sum( repmat(loss,[3 1]) .* cross( R*r, FF ), 2 ); % contact torque on base frame
%     F = sum(FF, 2 ); % contact force on base frame
%     T = sum(cross( R*r, FF ), 2 ); % contact torque on base frame
else
    F=[0 0 0]';
    T=[0 0 0]';
end

== matlab function pid_tv_test2/Gait Emulator/Walkway & force plate/FP Contact/MATLAB Function ==
  data: p input; F output; v input; Q input; w input; T output
function [F, T] = fcn(p, v, Q, w)
%#codegen

% if abs(p(1))<=0.25 && p(3)<=5e-3
if abs(p(1))<=0.25

% R = quat2dcm(Q);
R = [1 - 2*Q(3)^2 - 2*Q(4)^2	2*Q(2)*Q(3) - 2*Q(4)*Q(1)	2*Q(2)*Q(4) + 2*Q(3)*Q(1)
     2*Q(2)*Q(3) + 2*Q(4)*Q(1)	1 - 2*Q(2)^2 - 2*Q(4)^2	2*Q(3)*Q(4) - 2*Q(2)*Q(1)
     2*Q(2)*Q(4) - 2*Q(3)*Q(1)	2*Q(3)*Q(4) + 2*Q(2)*Q(1)	1 - 2*Q(2)^2 - 2*Q(3)^2];

th1 = linspace(-pi/2,pi/2,5);
% th1 = -pi/2 : 0.7 : pi/2;
r1 = 47e-3.*[cos(th1) cos(th1); sin(th1) sin(th1); zeros(size(th1)), zeros(size(th1))]; % circle
th2 = linspace(pi/2,-pi/2,5);
% th2 = pi/2 : -0.7 : -pi/2;
r2 = 47e-3.*[-cos(th2) -cos(th2); sin(th2) sin(th2); zeros(size(th2)), zeros(size(th2))]; % circle
r2(1,:) = bsxfun(@minus,r2(1,:),134e-3);
% r = ([1 1 1; 1 1 -1; 1 -1 1; 1 -1 -1; -1 1 1; -1 1 -1; -1 -1 1; -1 -1 -1].*repmat([0.2 0.1 0],8,1).*0.5).';
% xx = linspace(-0.11,-0.03,3);
xx = -0.07;
% xx = -0.12:0.04:-0.02;
r3 = [repmat(xx,1,2);repmat(47e-3,1,length(xx)),repmat(-47e-3,1,length(xx));zeros(1,size(xx,2)*2)];
r = [r1,r2,r3];

% spring-damper contact modelc
K = [0 0 0; 0 0 0; 0 0 1]*2e5;
B = [1 0 0; 0 1 0; 0 0 1]*2e3;
% K = [0 0 0; 0 0 0; 0 0 1]*2e4;
% B = [1 0 0; 0 1 0; 0 0 1]*2e2;

rr = bsxfun(@plus, R*r, p); % vertex position on base frame
vv = bsxfun(@plus, v, bsxfun(@cross, w, R*r)); % vertex velocity on base frame

FF = -K*(rr - 0) - B*vv; % force on vertex on base frame

% point is active if normal force is compressing ground
loss = 1 ./ ( 1 + exp(-[0.09 0.09 0.25]*FF) );
% loss = 1 ./ ( 1 + exp(150*[0 0 1]*rr) );

% displace force to coordinate center

% if abs(p(1))>=0.15 && abs(p(2))>=0.1
%     F=[0 0 0]';
%     T=[0 0 0]';
% else
%     if any(rr(3,:)) && mean(nonzeros(rr(3,:)))<=5e-3
%     if any(rr(3,:)<=5e-3)
        F = sum( repmat(loss,[3 1]) .* FF, 2 ); % contact force on base frame
        T = sum( repmat(loss,[3 1]) .* cross( R*r, FF ), 2 ); % contact torque on base frame
%     else
%         F=[0 0 0]';
%         T=[0 0 0]';
%     end
%     F = sum(FF, 2 ); % contact force on base frame
%     T = sum(cross( R*r, FF ), 2 ); % contact torque on base frame
else
    F=[0 0 0]';
    T=[0 0 0]';
end

== matlab function pid_tv_test2/MATLAB Function1 ==
  data: t input; q input; qp output; dev output
function [qp, dev] = ik_sol(t, q)
%#codegen
[qp, dev] = ik_test(t, q/2);
